simulink model "chap7_6sim"  (Simulink 8.1)
settings: Solver=ode45  StartTime=0.0  StopTime=50  FixedStep=0.001  RelTol=1e-3
settings Model: Creator=liujk  LastModifiedBy=liujk  ExtModeTrigMode=oneshot  ExtModeArmWhenConnect=off
settings DataIOCC: LimitDataPoints=off  SignalLoggingName=sigsOut
settings OptimizationCC: BooleanDataType=off  ExpressionDepthLimit=128  InitFltsAndDblsToZero=on
settings DebuggingCC: SaveWithParameterizedLinksMsg=none  SignalResolutionControl=TryResolveAllWithWarning  SolverPrmCheckMsg=none  MultiTaskDSMMsg=warning  MultiTaskCondExecSysMsg=none  StrictBusMsg=None
settings HardwareCC: TargetUnknown=on
settings RTWCC: IncludeERTFirstTime=on
settings GRTTargetCC: TargetFcnLib=ansi_tfl_tmw.mat

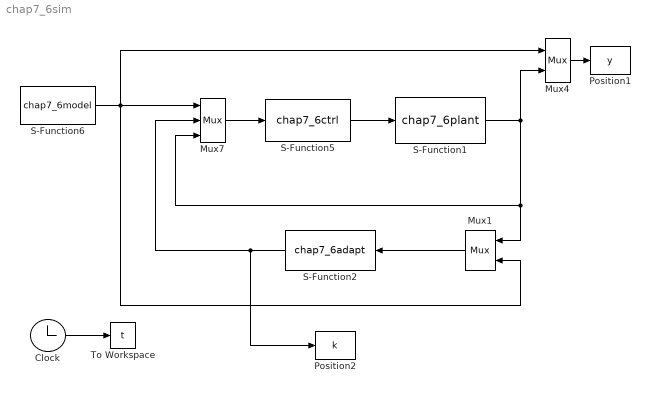
== system chap7_6sim ==
  Clock : Clock
  Mux1 : Mux  Inputs=2
  Mux4 : Mux  Inputs=2
  Mux7 : Mux  Inputs=3
  Position1 : ToWorkspace  VariableName=y  SampleTime=-1
  Position2 : ToWorkspace  VariableName=k  SampleTime=-1
  S-Function1 : S-Function  FunctionName=chap7_6plant  EnableBusSupport=off
  S-Function2 : S-Function  FunctionName=chap7_6adapt  EnableBusSupport=off
  S-Function5 : S-Function  FunctionName=chap7_6ctrl  EnableBusSupport=off
  S-Function6 : S-Function  FunctionName=chap7_6model  EnableBusSupport=off
  To Workspace : ToWorkspace  VariableName=t  SampleTime=-1
  wires:
  Clock/1 -> To Workspace/1
  S-Function6/1 -> Mux7/1, Mux4/1, Mux1/2
  S-Function1/1 -> Mux4/2, Mux7/3, Mux1/1
  S-Function5/1 -> S-Function1/1
  Mux4/1 -> Position1/1
  Mux7/1 -> S-Function5/1
  S-Function2/1 -> Mux7/2, Position2/1
  Mux1/1 -> S-Function2/1
